simulink model "main"  (R2021a)
settings: Solver=VariableStepAuto  StartTime=0.0  StopTime=10  RelTol=1e-3
libraries: dsparch4 x20, dspsrcs4 x20
settings Model: Creator=Bharat Gunhalkar  LastModifiedBy=Bharat Gunhalkar

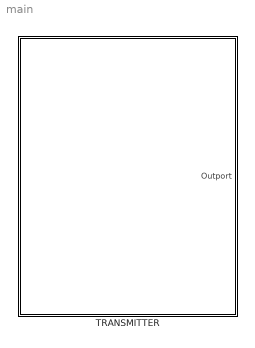
== system main ==
  TRANSMITTER : Subsystem

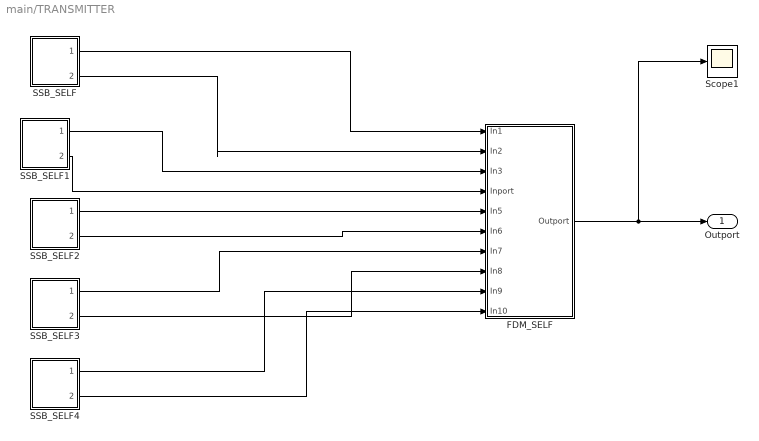
== system main/TRANSMITTER ==
  FDM_SELF : Subsystem
  SSB_SELF : Subsystem
  SSB_SELF1 : Subsystem
  SSB_SELF2 : Subsystem
  SSB_SELF3 : Subsystem
  SSB_SELF4 : Subsystem
  Scope1 : Scope
  Outport : Outport
  wires:
  SSB_SELF4/1(Outport) -> FDM_SELF/9(In9)
  SSB_SELF4/2(Outport1) -> FDM_SELF/10(In10)
  SSB_SELF1/1(Outport) -> FDM_SELF/3(In3)
  SSB_SELF3/1(Outport) -> FDM_SELF/7(In7)
  SSB_SELF2/1(Outport) -> FDM_SELF/5(In5)
  SSB_SELF2/2(Outport1) -> FDM_SELF/6(In6)
  FDM_SELF/1(Outport) -> Outport/1, Scope1/1
  SSB_SELF/1(Outport) -> FDM_SELF/1(In1)
  SSB_SELF/2(Outport1) -> FDM_SELF/2(In2)
  SSB_SELF3/2(Outport1) -> FDM_SELF/8(In8)
  SSB_SELF1/2(Outport1) -> FDM_SELF/4(Inport)

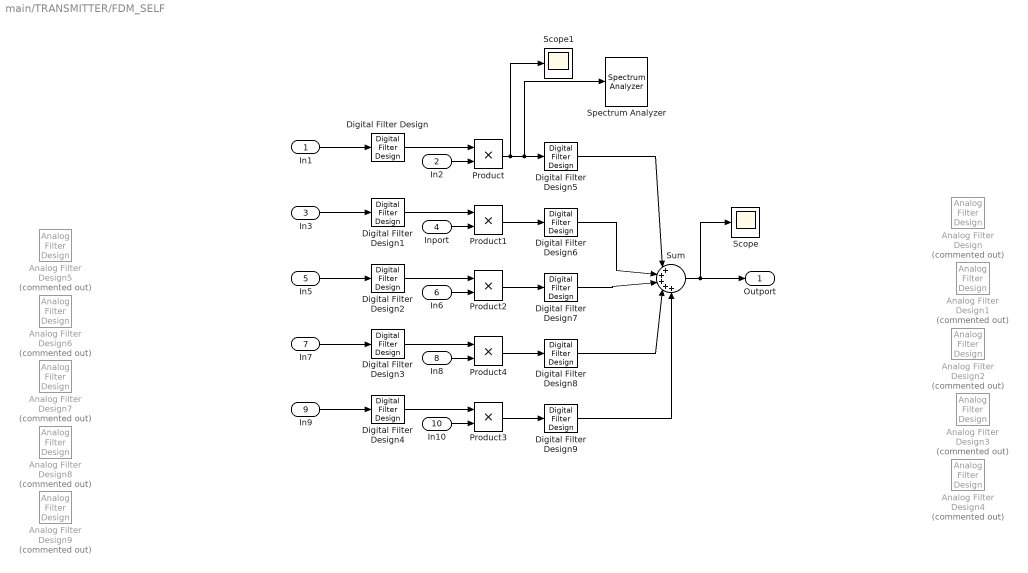
== system main/TRANSMITTER/FDM_SELF ==
  In1 : Inport
  In2 : Inport  Port=2
  In3 : Inport  Port=3
  Inport : Inport  Port=4
  In5 : Inport  Port=5
  In6 : Inport  Port=6
  In7 : Inport  Port=7
  In8 : Inport  Port=8
  In9 : Inport  Port=9
  In10 : Inport  Port=10
  Analog Filter Design{,1..4} (5 alike) : dsparch4/Analog Filter Design  Commented=on  method=Butterworth  filttype=Lowpass  N=8  Wlo=30  Whi=80  Rp=2  Rs=40
  Analog Filter Design{5..9} (5 alike) : dsparch4/Analog Filter Design  Commented=on  method=Butterworth  filttype=Bandpass  N=8  Wlo=30  Whi=80  Rp=2  Rs=40
  Digital Filter Design{,1..9} (10 alike) : dsparch4/Digital Filter Design  mwdsp_browser_bugfix_var=off
  Product{,1..4} (5 alike) : Product
  Scope : Scope
  Scope1 : Scope
  Spectrum Analyzer : SpectrumAnalyzer
  Sum : Sum  Inputs=|+++++
  Outport : Outport
  wires:
  In3/1 -> Digital Filter Design1/1
  Digital Filter Design2/1 -> Product2/1
  Digital Filter Design6/1 -> Sum/2
  In5/1 -> Digital Filter Design2/1
  Digital Filter Design5/1 -> Sum/1
  Digital Filter Design3/1 -> Product4/1
  Digital Filter Design9/1 -> Sum/5
  Digital Filter Design1/1 -> Product1/1
  Product3/1 -> Digital Filter Design9/1
  In7/1 -> Digital Filter Design3/1
  Product/1 -> Scope1/1, Spectrum Analyzer/1, Digital Filter Design5/1
  Digital Filter Design/1 -> Product/1
  Product1/1 -> Digital Filter Design6/1
  Digital Filter Design8/1 -> Sum/4
  Digital Filter Design4/1 -> Product3/1
  In6/1 -> Product2/2
  Sum/1 -> Outport/1, Scope/1
  Product2/1 -> Digital Filter Design7/1
  Digital Filter Design7/1 -> Sum/3
  In2/1 -> Product/2
  In8/1 -> Product4/2
  In10/1 -> Product3/2
  Product4/1 -> Digital Filter Design8/1
  In1/1 -> Digital Filter Design/1
  In9/1 -> Digital Filter Design4/1
  Inport/1 -> Product1/2

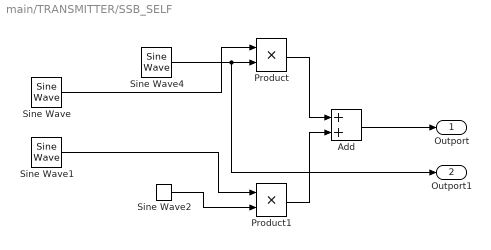
== system main/TRANSMITTER/SSB_SELF ==
  Add : Sum
  Product : Product
  Product1 : Product
  Sine Wave : dspsrcs4/Sine Wave  Amplitude=1  Frequency=100  Phase=0  SampleMode=Discrete  OutComplex=Real  CompMethod=Trigonometric fcn  TableSize=Speed  SampleTime=1/20000  SamplesPerFrame=1  ResetState=Restart at time zero  OutputFrames=off  dataType=double  wordLen=16  udDataType=sfix(16)  fracBitsMode=Best precision  numFracBits=15  OutDataTypeStr=double  LastOutDataTypeStr=double
  Sine Wave1 : dspsrcs4/Sine Wave  Amplitude=1  Frequency=100  Phase=-(pi/2)  SampleMode=Discrete  OutComplex=Real  CompMethod=Trigonometric fcn  TableSize=Speed  SampleTime=1/20000  SamplesPerFrame=1  ResetState=Restart at time zero  OutputFrames=off  dataType=double  wordLen=16  udDataType=sfix(16)  fracBitsMode=Best precision  numFracBits=15  OutDataTypeStr=double  LastOutDataTypeStr=double
  Sine Wave2 : dspsrcs4/Sine Wave  Amplitude=1  Frequency=1000  Phase=-(pi/2)  SampleMode=Discrete  OutComplex=Real  CompMethod=Trigonometric fcn  TableSize=Speed  SampleTime=1/20000  SamplesPerFrame=1  ResetState=Restart at time zero  OutputFrames=off  dataType=double  wordLen=16  udDataType=sfix(16)  fracBitsMode=Best precision  numFracBits=15  OutDataTypeStr=double  LastOutDataTypeStr=double
  Sine Wave4 : dspsrcs4/Sine Wave  Amplitude=1  Frequency=1000  Phase=0  SampleMode=Discrete  OutComplex=Real  CompMethod=Trigonometric fcn  TableSize=Speed  SampleTime=1/20000  SamplesPerFrame=1  ResetState=Restart at time zero  OutputFrames=off  dataType=double  wordLen=16  udDataType=sfix(16)  fracBitsMode=Best precision  numFracBits=15  OutDataTypeStr=double  LastOutDataTypeStr=double
  Outport : Outport
  Outport1 : Outport  Port=2
  wires:
  Product/1 -> Add/1
  Product1/1 -> Add/2
  Sine Wave2/1 -> Product1/2
  Sine Wave/1 -> Product/1
  Sine Wave4/1 -> Outport1/1, Product/2
  Sine Wave1/1 -> Product1/1
  Add/1 -> Outport/1

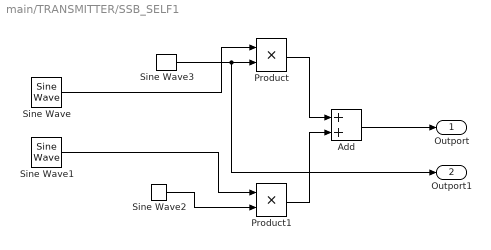
== system main/TRANSMITTER/SSB_SELF1 ==
  Add : Sum
  Product : Product
  Product1 : Product
  Sine Wave : dspsrcs4/Sine Wave  Amplitude=1  Frequency=200  Phase=0  SampleMode=Discrete  OutComplex=Real  CompMethod=Trigonometric fcn  TableSize=Speed  SampleTime=1/20000  SamplesPerFrame=1  ResetState=Restart at time zero  OutputFrames=off  dataType=double  wordLen=16  udDataType=sfix(16)  fracBitsMode=Best precision  numFracBits=15  OutDataTypeStr=double  LastOutDataTypeStr=double
  Sine Wave1 : dspsrcs4/Sine Wave  Amplitude=1  Frequency=200  Phase=-(pi/2)  SampleMode=Discrete  OutComplex=Real  CompMethod=Trigonometric fcn  TableSize=Speed  SampleTime=1/20000  SamplesPerFrame=1  ResetState=Restart at time zero  OutputFrames=off  dataType=double  wordLen=16  udDataType=sfix(16)  fracBitsMode=Best precision  numFracBits=15  OutDataTypeStr=double  LastOutDataTypeStr=double
  Sine Wave2 : dspsrcs4/Sine Wave  Amplitude=1  Frequency=1000  Phase=-(pi/2)  SampleMode=Discrete  OutComplex=Real  CompMethod=Trigonometric fcn  TableSize=Speed  SampleTime=1/20000  SamplesPerFrame=1  ResetState=Restart at time zero  OutputFrames=off  dataType=double  wordLen=16  udDataType=sfix(16)  fracBitsMode=Best precision  numFracBits=15  OutDataTypeStr=double  LastOutDataTypeStr=double
  Sine Wave3 : dspsrcs4/Sine Wave  Amplitude=1  Frequency=1000  Phase=0  SampleMode=Discrete  OutComplex=Real  CompMethod=Trigonometric fcn  TableSize=Speed  SampleTime=1/20000  SamplesPerFrame=1  ResetState=Restart at time zero  OutputFrames=off  dataType=double  wordLen=16  udDataType=sfix(16)  fracBitsMode=Best precision  numFracBits=15  OutDataTypeStr=double  LastOutDataTypeStr=double
  Outport : Outport
  Outport1 : Outport  Port=2
  wires:
  Product/1 -> Add/1
  Product1/1 -> Add/2
  Sine Wave2/1 -> Product1/2
  Sine Wave/1 -> Product/1
  Sine Wave3/1 -> Outport1/1, Product/2
  Sine Wave1/1 -> Product1/1
  Add/1 -> Outport/1

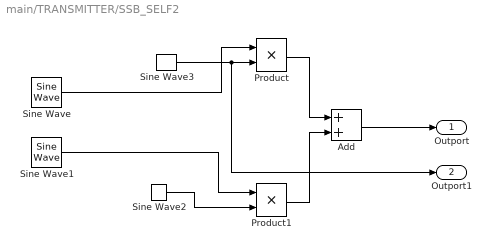
== system main/TRANSMITTER/SSB_SELF2 ==
  Add : Sum
  Product : Product
  Product1 : Product
  Sine Wave : dspsrcs4/Sine Wave  Amplitude=1  Frequency=300  Phase=0  SampleMode=Discrete  OutComplex=Real  CompMethod=Trigonometric fcn  TableSize=Speed  SampleTime=1/20000  SamplesPerFrame=1  ResetState=Restart at time zero  OutputFrames=off  dataType=double  wordLen=16  udDataType=sfix(16)  fracBitsMode=Best precision  numFracBits=15  OutDataTypeStr=double  LastOutDataTypeStr=double
  Sine Wave1 : dspsrcs4/Sine Wave  Amplitude=1  Frequency=300  Phase=-(pi/2)  SampleMode=Discrete  OutComplex=Real  CompMethod=Trigonometric fcn  TableSize=Speed  SampleTime=1/20000  SamplesPerFrame=1  ResetState=Restart at time zero  OutputFrames=off  dataType=double  wordLen=16  udDataType=sfix(16)  fracBitsMode=Best precision  numFracBits=15  OutDataTypeStr=double  LastOutDataTypeStr=double
  Sine Wave2 : dspsrcs4/Sine Wave  Amplitude=1  Frequency=1000  Phase=-(pi/2)  SampleMode=Discrete  OutComplex=Real  CompMethod=Trigonometric fcn  TableSize=Speed  SampleTime=1/20000  SamplesPerFrame=1  ResetState=Restart at time zero  OutputFrames=off  dataType=double  wordLen=16  udDataType=sfix(16)  fracBitsMode=Best precision  numFracBits=15  OutDataTypeStr=double  LastOutDataTypeStr=double
  Sine Wave3 : dspsrcs4/Sine Wave  Amplitude=1  Frequency=1000  Phase=0  SampleMode=Discrete  OutComplex=Real  CompMethod=Trigonometric fcn  TableSize=Speed  SampleTime=1/20000  SamplesPerFrame=1  ResetState=Restart at time zero  OutputFrames=off  dataType=double  wordLen=16  udDataType=sfix(16)  fracBitsMode=Best precision  numFracBits=15  OutDataTypeStr=double  LastOutDataTypeStr=double
  Outport : Outport
  Outport1 : Outport  Port=2
  wires:
  Product/1 -> Add/1
  Product1/1 -> Add/2
  Sine Wave2/1 -> Product1/2
  Sine Wave/1 -> Product/1
  Sine Wave3/1 -> Outport1/1, Product/2
  Sine Wave1/1 -> Product1/1
  Add/1 -> Outport/1

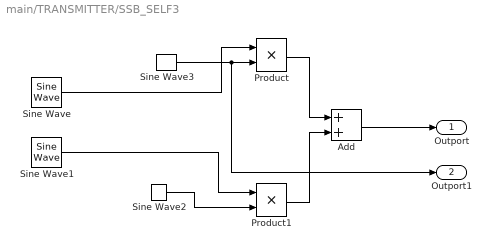
== system main/TRANSMITTER/SSB_SELF3 ==
  Add : Sum
  Product : Product
  Product1 : Product
  Sine Wave : dspsrcs4/Sine Wave  Amplitude=1  Frequency=400  Phase=0  SampleMode=Discrete  OutComplex=Real  CompMethod=Trigonometric fcn  TableSize=Speed  SampleTime=1/20000  SamplesPerFrame=1  ResetState=Restart at time zero  OutputFrames=off  dataType=double  wordLen=16  udDataType=sfix(16)  fracBitsMode=Best precision  numFracBits=15  OutDataTypeStr=double  LastOutDataTypeStr=double
  Sine Wave1 : dspsrcs4/Sine Wave  Amplitude=1  Frequency=400  Phase=-(pi/2)  SampleMode=Discrete  OutComplex=Real  CompMethod=Trigonometric fcn  TableSize=Speed  SampleTime=1/20000  SamplesPerFrame=1  ResetState=Restart at time zero  OutputFrames=off  dataType=double  wordLen=16  udDataType=sfix(16)  fracBitsMode=Best precision  numFracBits=15  OutDataTypeStr=double  LastOutDataTypeStr=double
  Sine Wave2 : dspsrcs4/Sine Wave  Amplitude=1  Frequency=1000  Phase=-(pi/2)  SampleMode=Discrete  OutComplex=Real  CompMethod=Trigonometric fcn  TableSize=Speed  SampleTime=1/20000  SamplesPerFrame=1  ResetState=Restart at time zero  OutputFrames=off  dataType=double  wordLen=16  udDataType=sfix(16)  fracBitsMode=Best precision  numFracBits=15  OutDataTypeStr=double  LastOutDataTypeStr=double
  Sine Wave3 : dspsrcs4/Sine Wave  Amplitude=1  Frequency=1000  Phase=0  SampleMode=Discrete  OutComplex=Real  CompMethod=Trigonometric fcn  TableSize=Speed  SampleTime=1/20000  SamplesPerFrame=1  ResetState=Restart at time zero  OutputFrames=off  dataType=double  wordLen=16  udDataType=sfix(16)  fracBitsMode=Best precision  numFracBits=15  OutDataTypeStr=double  LastOutDataTypeStr=double
  Outport : Outport
  Outport1 : Outport  Port=2
  wires:
  Product/1 -> Add/1
  Product1/1 -> Add/2
  Sine Wave2/1 -> Product1/2
  Sine Wave/1 -> Product/1
  Sine Wave3/1 -> Outport1/1, Product/2
  Sine Wave1/1 -> Product1/1
  Add/1 -> Outport/1

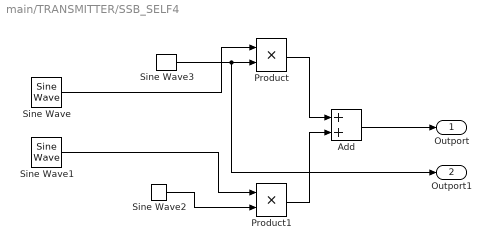
== system main/TRANSMITTER/SSB_SELF4 ==
  Add : Sum
  Product : Product
  Product1 : Product
  Sine Wave : dspsrcs4/Sine Wave  Amplitude=1  Frequency=500  Phase=0  SampleMode=Discrete  OutComplex=Real  CompMethod=Trigonometric fcn  TableSize=Speed  SampleTime=1/20000  SamplesPerFrame=1  ResetState=Restart at time zero  OutputFrames=off  dataType=double  wordLen=16  udDataType=sfix(16)  fracBitsMode=Best precision  numFracBits=15  OutDataTypeStr=double  LastOutDataTypeStr=double
  Sine Wave1 : dspsrcs4/Sine Wave  Amplitude=1  Frequency=500  Phase=-(pi/2)  SampleMode=Discrete  OutComplex=Real  CompMethod=Trigonometric fcn  TableSize=Speed  SampleTime=1/20000  SamplesPerFrame=1  ResetState=Restart at time zero  OutputFrames=off  dataType=double  wordLen=16  udDataType=sfix(16)  fracBitsMode=Best precision  numFracBits=15  OutDataTypeStr=double  LastOutDataTypeStr=double
  Sine Wave2 : dspsrcs4/Sine Wave  Amplitude=1  Frequency=1000  Phase=-(pi/2)  SampleMode=Discrete  OutComplex=Real  CompMethod=Trigonometric fcn  TableSize=Speed  SampleTime=1/20000  SamplesPerFrame=1  ResetState=Restart at time zero  OutputFrames=off  dataType=double  wordLen=16  udDataType=sfix(16)  fracBitsMode=Best precision  numFracBits=15  OutDataTypeStr=double  LastOutDataTypeStr=double
  Sine Wave3 : dspsrcs4/Sine Wave  Amplitude=1  Frequency=1000  Phase=0  SampleMode=Discrete  OutComplex=Real  CompMethod=Trigonometric fcn  TableSize=Speed  SampleTime=1/20000  SamplesPerFrame=1  ResetState=Restart at time zero  OutputFrames=off  dataType=double  wordLen=16  udDataType=sfix(16)  fracBitsMode=Best precision  numFracBits=15  OutDataTypeStr=double  LastOutDataTypeStr=double
  Outport : Outport
  Outport1 : Outport  Port=2
  wires:
  Product/1 -> Add/1
  Product1/1 -> Add/2
  Sine Wave2/1 -> Product1/2
  Sine Wave/1 -> Product/1
  Sine Wave3/1 -> Outport1/1, Product/2
  Sine Wave1/1 -> Product1/1
  Add/1 -> Outport/1
